simulink model "DatacenterUtilization"  (R2025b)
settings: Solver=daessc  StartTime=0.0  StopTime=7776000  FixedStep=3600  MaxStep=3600  RelTol=1e-3  AbsTol=1e-3
undefined symbols (not defined in the file or in its folder): Datacenter, MyDatacenterModelLib, Room
libraries: fl_lib x111, buildingEnergy_lib x13, datacenter_lib x12, nesl_utility x5
settings Model: Creator=vikrants  LastModifiedBy=skota
settings SolverCC: AutoScaleAbsTol=off  AlgebraicLoopSolver=TrustRegion  MaxZcPerStep=1.0
settings DataIOCC: SaveOutput=off  SignalLogging=off  DSMLogging=off  SaveTime=off  ReturnWorkspaceOutputs=off  TimeSaveName=tSim  SignalLoggingName=sglDatacenterUtilization  ReturnWorkspaceOutputsName=resDatacenterUtilization
settings DebuggingCC: UnconnectedInputMsg=warning  UnconnectedOutputMsg=warning  UnconnectedLineMsg=warning  SymbolicDimsDataTypeCodeGenerationDiagnostic=none
settings ModelReferenceCC: EnableRefExpFcnMdlSchedulingChecks=on
settings SFSimCC: CustomCodeUndefinedFunction=UseInterfaceOnly
settings RTWCC: GPUComputeCapability=3.5  DLArmComputeVersion=19.05
settings SimscapeCC: SimscapeLogType=all  SimscapeLogName=simlogDatacenterUtilization  SimscapeLogLimitData=off  SimscapeLogDataHistory=10000.0  SimscapeCompileComponentReuse=on

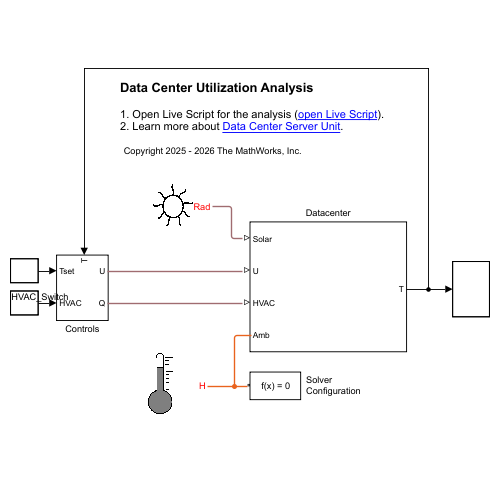
[thumbnail: Simulink's stored preview of the top-level diagram]
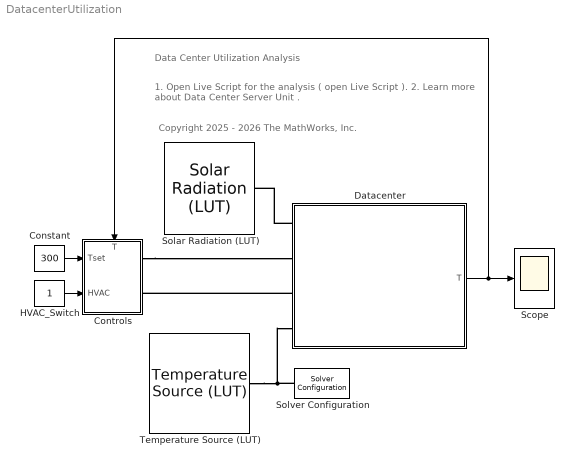
== system DatacenterUtilization ==
  note: Copyright 2025 - 2026 The MathWorks, Inc.
  note: Data Center Utilization Analysis
  note: 1. Open Live Script for the analysis ( open Live Script ).
      | 2. Learn more about Data Center Server Unit .
  Constant : Constant  Value=300
  Controls : Subsystem
      settings: PortSchema="{\"entries\":[{\"content\":{\"sides\":[{\"content\":{\"connectorIds\":[\"In1\",\"In2\"]},\"type\":\"ConnectorPlacement.EquallySpacedRectSide\",\"uuid\":\"920383aa-55f0-46ec-be25-1a0e41e599a9\"},{\"content\":{\"connectorIds\":[\"RConn1\",\"RConn2\"],\"side\":\"RIGHT\"},\"type\":\"ConnectorPlacement.EquallySpacedRectSide\",\"uuid\":\"2611bc07-e966-40b9-ba68-b41ec292afae\"},{\"content\":{\"connectorIds\":[\"In3\"],\"side\":\"TOP\"},\"type\":\"ConnectorPlacement.EquallySpacedRectSide\",\"uuid\":\"ac1e2822-ea25-44fd-bd61-5e24e36934cf\"}]},\"type\":\"ConnectorPlacement.EquallySpacedConnector\",\"uuid\":\"6950ab52-c187-4a89-be73-f973560319f4\"}],\"packageUris\":[\"http://schema.mathworks.com/mf0/Connector/R2020b\"],\"version\":\"1.0\"}"
  Datacenter : Subsystem
  HVAC_Switch : Constant
  Scope : Scope
      settings: ActiveDisplayYMinimum=298.50227589858127  ActiveDisplayYMaximum=313.47951691276859
  Solar Radiation (LUT) : buildingEnergy_lib/Solar Radiation (LUT)  latitude=12.971 % Parameterized on : 26-May-2026 12:20:46  longitude=77.594 % Parameterized on : 26-May-2026 12:20:46  localTime=82.5 % Parameterized on : 26-May-2026 12:20:46  dayLightS=0 % Parameterized on : 26-May-2026 12:20:46  startYear=2025 % Parameterized on : 26-May-2026 12:20:46  startMonth=1 % Parameterized on : 26-May-2026 12:20:46  startDay=1 % Parameterized on : 26-May-2026 12:20:46  startHr=1 % Parameterized on : 26-May-2026 12:20:46  numHrsData=2160 % Parameterized on : 26-May-2026 12:20:46  cloudData=cloudCoverLibOption.none  cloudCoverVal=zeros(1, 24)  interp_method=simscape.enum.interpolation.linear  extrap_method=simscape.enum.extrapolation.nearest
  Solver Configuration : nesl_utility/Solver Configuration  PhysicalDomain=network_engine_domain  SubClassName=solver  LeftPortType=input  RightPortType=generic  Tones=[]  Harmonics=[]  SimulateNoise=off  Profile=off  UseLocalSampling=off  EnableSwitchedLinearOptims=on  FrequencyDomain=off  UseCCode=off  RelTol=0.001  AbsTol=1e-06  MinStep=1e-09  ToWorkspace=off  RevertToSquareIcSolve=off  NumHomotopyIterations=100  PhasorMode=off  PhasorModeNumHarmonics=1  ConsistencySolver=NEWTON_XTOL_AFTER_FTOL  CanonicalOrdering=UNORDERED  OptimizeIntermediates=UNOPTIMIZED  IndexReductionMethod=DerivativeReplacement  DoDC=off  ResidualTolerance=1e-09  ConsistencyTolSource=GLOBAL  ConsistencyAbsTol=0.001  ConsistencyRelTol=0.001  ConsistencyTolFactor=0.001  UseLocalSolver=off  LocalSolverChoice=NE_BACKWARD_EULER_ADVANCER  ResolveIndetEquations=on  FunctionEvalNumThread=1  LocalSolverSampleTime=0.001  DoFixedCost=off  MaxNonlinIter=3  MaxModeIter=2  ComputeImpulses=off  ImpulseIterations=2  LinearAlgebra=auto  LinearAlgebraNumThread=0  EquationFormulation=NE_TIME_EF  DelaysMemoryBudget=1024  AutomaticFiltering=on  FilteringTimeConstant=0.001  PartitionStorageMethod=AS_NEEDED  PartitionMemoryBudget=1024  PartitionMethod=ROBUST  MultibodyUseLocalSolver=off  MultibodyLocalSolverChoice=ODE1  MultibodyLocalSolverSampleTime=0.001
  Temperature Source (LUT) : buildingEnergy_lib/Temperature Source (LUT)  latitude=12.971 % Parameterized on : 26-May-2026 12:20:45  longitude=77.594 % Parameterized on : 26-May-2026 12:20:45  localTime=82.5 % Parameterized on : 26-May-2026 12:20:45  dayLightS=0 % Parameterized on : 26-May-2026 12:20:46  startYear=2025 % Parameterized on : 26-May-2026 12:20:46  startMonth=1 % Parameterized on : 26-May-2026 12:20:46  startDay=1 % Parameterized on : 26-May-2026 12:20:46  startHr=1 % Parameterized on : 26-May-2026 12:20:46  numDaysData=91 % Parameterized on : 26-May-2026 12:20:46  interp_method=simscape.enum.interpolation.linear  extrap_method=simscape.enum.extrapolation.error  avgDayTvec=[309 309 309 309 309 309 309 309 309 309 309 309 309 309 309 309 309 309 309 309 309 309 309 309 309 309 309 309 309 309 309 309 309 309 309 309 309 309 309 309 309 309 309 309 309 309 309 309 309 309 309 309 309 309 309 309 309 309 309 309 309 309 309 309 309 309 309 309 309 309 309 309 309 309 309 309 309 309 309 309 309 309 309 309 309 309 309 309 309 309 309] K  pcDayTvar=5  avgNightTvec=[301 301 301 301 301 301 301 301 301 301 301 301 301 301 301 301 301 301 301 301 301 301 301 301 301 301 301 301 301 301 301 301 301 301 301 301 301 301 301 301 301 301 301 301 301 301 301 301 301 301 301 301 301 301 301 301 301 301 301 301 301 301 301 301 301 301 301 301 301 301 301 301 301 301 301 301 301 301 301 301 301 301 301 301 301 301 301 301 301 301 301] K  pcNightTvar=5
  wires:
  Constant/1 -> Controls/1(Tset)
  Datacenter/1(T) -> Scope/1, Controls/3(T)
  HVAC_Switch/1 -> Controls/2(HVAC)
  connections:
  Solver Configuration/RConn1 -- Temperature Source (LUT)/RConn1 -- Datacenter/LConn4
  Datacenter/LConn3 -- Controls/RConn2
  Datacenter/LConn1 -- Solar Radiation (LUT)/RConn1
  Controls/RConn1 -- Datacenter/LConn2

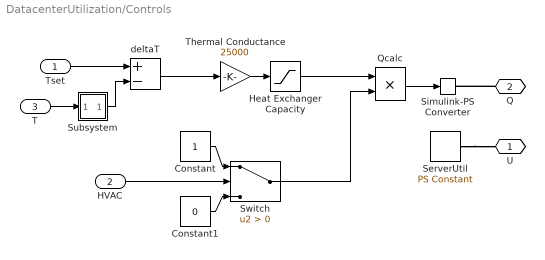
== system DatacenterUtilization/Controls ==
  Tset : Inport
  HVAC : Inport  Port=2
  T : Inport  Port=3
  Constant : Constant
  Constant1 : Constant  Value=0
  Heat Exchanger Capacity : Saturate  UpperLimit=100000  LowerLimit=-100000
  Qcalc : Product
  ServerUtil : fl_lib/Physical Signals/Sources/PS Constant  constant=[0.48 0.42 0.45 0.51 0.52 0.58 0.37 0.33 0.39 0.44 0.41 0.41]
  Simulink-PS Converter : nesl_utility/Simulink-PS Converter  PhysicalDomain=network_engine_domain  SubClassName=ps_input  LeftPortType=input  RightPortType=output  PseudoPeriodic=off  Frequencies=[]  NoiseDistribution=none  NoiseParameters=[]  Unit=W  AffineConversion=off  FilteringAndDerivatives=provide  SimscapeFilterOrder=1  InputFilterTimeConstant=0.001  UdotUserProvided=0
  Subsystem : Subsystem
  Switch : Switch  Criteria=u2 > Threshold  SaturateOnIntegerOverflow=off  InputSameDT=off
  Thermal Conductance : Gain  Gain=25000
  deltaT : Sum  Inputs=+-
  U : PMIOPort  Side=Right
  Q : PMIOPort  Port=2  Side=Right
  wires:
  Tset/1 -> deltaT/1
  HVAC/1 -> Switch/2
  Constant/1 -> Switch/1
  Constant1/1 -> Switch/3
  Switch/1 -> Qcalc/2
  Qcalc/1 -> Simulink-PS Converter/1
  deltaT/1 -> Thermal Conductance/1
  Thermal Conductance/1 -> Heat Exchanger Capacity/1
  Heat Exchanger Capacity/1 -> Qcalc/1
  T/1 -> Subsystem/1("  ")
  Subsystem/1(" ") -> deltaT/2
  connections:
  Q/RConn1 -- Simulink-PS Converter/RConn1
  ServerUtil/RConn1 -- U/RConn1

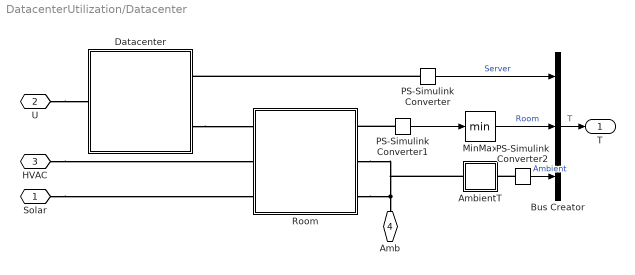
== system DatacenterUtilization/Datacenter ==
  AmbientT : Subsystem
  Bus Creator : BusCreator  Inputs=3
  Datacenter : Subsystem  AncestorBlock=MyDatacenterModelLib/Datacenter
  MinMax : MinMax
  PS-Simulink Converter : nesl_utility/PS-Simulink Converter  PhysicalDomain=network_engine_domain  SubClassName=ps_output  LeftPortType=input  RightPortType=output  PseudoPeriodic=off  Frequencies=[]  VectorFormat=inherit  Unit=inherit  AffineConversion=off
  PS-Simulink Converter1 : nesl_utility/PS-Simulink Converter  PhysicalDomain=network_engine_domain  SubClassName=ps_output  LeftPortType=input  RightPortType=output  PseudoPeriodic=off  Frequencies=[]  VectorFormat=inherit  Unit=inherit  AffineConversion=off
  PS-Simulink Converter2 : nesl_utility/PS-Simulink Converter  PhysicalDomain=network_engine_domain  SubClassName=ps_output  LeftPortType=input  RightPortType=output  PseudoPeriodic=off  Frequencies=[]  VectorFormat=inherit  Unit=inherit  AffineConversion=off
  Room : Subsystem  AncestorBlock=MyDatacenterModelLib/Room
  Solar : PMIOPort  Side=Left
  U : PMIOPort  Port=2  Side=Left
  HVAC : PMIOPort  Port=3  Side=Left
  Amb : PMIOPort  Port=4  Side=Left
  T : Outport
  wires:
  Bus Creator/1 -> T/1  "T"
  PS-Simulink Converter2/1 -> Bus Creator/3  "Ambient"
  PS-Simulink Converter1/1 -> MinMax/1
  PS-Simulink Converter/1 -> Bus Creator/1  "Server"
  MinMax/1 -> Bus Creator/2  "Room"
  connections:
  PS-Simulink Converter2/LConn1 -- AmbientT/RConn1
  Datacenter/RConn2 -- Room/LConn1
  U/RConn1 -- Datacenter/LConn1
  PS-Simulink Converter/LConn1 -- Datacenter/RConn1
  Room/RConn3 -- Room/RConn2 -- AmbientT/LConn1 -- Amb/RConn1
  PS-Simulink Converter1/LConn1 -- Room/RConn1
  HVAC/RConn1 -- Room/LConn2
  Solar/RConn1 -- Room/LConn3

== system DatacenterUtilization/Controls/Subsystem ==
  "  " : Inport
  Bus Selector1 : BusSelector  OutputSignals=Room
  Transfer Fcn : TransferFcn  Denominator=[1 1]
  " " : Outport
  wires:
  Bus Selector1/1 -> Transfer Fcn/1  "<Room>"
  "  "/1 -> Bus Selector1/1
  Transfer Fcn/1 -> " "/1

== system DatacenterUtilization/Datacenter/AmbientT ==
  Tref : fl_lib/Thermal/Thermal Elements/Thermal Reference
  Tsensor3 : fl_lib/Thermal/Thermal Sensors/Temperature Sensor  temperature_measure=foundation.enum.MeasurementReference.difference
  "   " : PMIOPort  Side=Left
  T : PMIOPort  Port=2  Side=Right
  connections:
  Tsensor3/RConn1 -- Tref/LConn1
  Tsensor3/RConn2 -- T/RConn1
  Tsensor3/LConn1 -- "   "/RConn1

== system DatacenterUtilization/Datacenter/Datacenter ==
  ServerUnits : Subsystem
  Util : PMIOPort  Side=Left
  T : PMIOPort  Port=2  Side=Right
  H : PMIOPort  Port=3  Side=Right
  connections:
  ServerUnits/RConn1 -- H/RConn1
  ServerUnits/RConn2 -- T/RConn1
  ServerUnits/LConn1 -- Util/RConn1

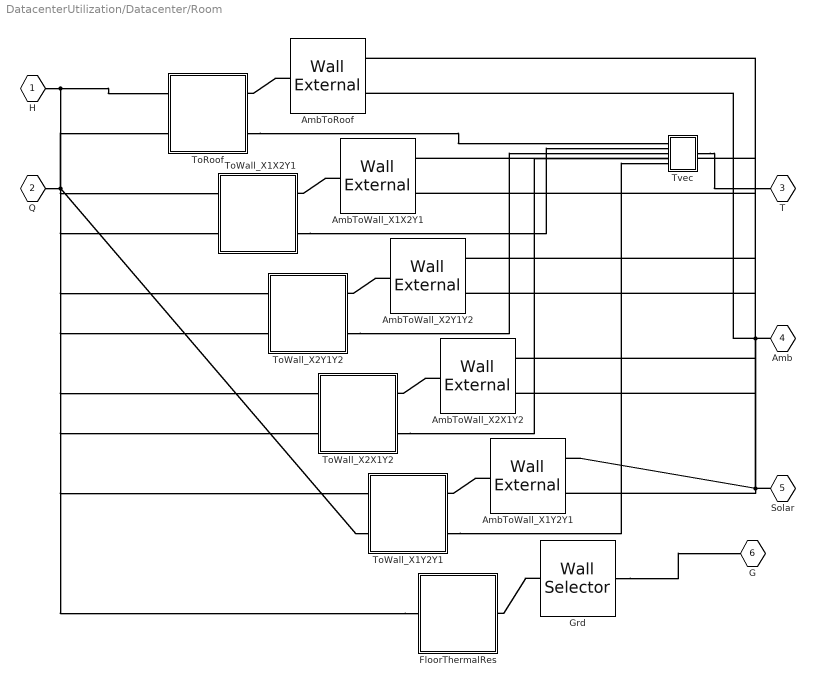
== system DatacenterUtilization/Datacenter/Room ==
  AmbToRoof : buildingEnergy_lib/Wall External  extWallModel=wallExternalModelOption.wallSolarWinVent  wallLength=12 m  wallHeight=8 m  wallThickness=0.05 m  wallMaterialDen=4000 kg/m^3  wallMaterialCp=1870 J/(K*kg)  wallAbsorptivity=0.5  wallThermalK=2 W/(K*m)  winLength=1 m  winHeight=0.5 m  winThickness=0.007 m  winMaterialDen=2500 kg/m^3  winMaterialCp=787 J/(K*kg)  winAbsorptivity=0.35  winThermalK=1 W/(K*m)  winTransmissivity=0.45  ventLength=0.1 m  ventHeight=0.1 m  extToWallHTC=5 W/(K*m^2)  intToRoomHTC=5 W/(K*m^2)  iniT=300 K  latitude=12.971 % Parameterized on : 26-May-2026 12:20:46  longitude=77.594 % Parameterized on : 26-May-2026 12:20:46  localTime=82.5 % Parameterized on : 26-May-2026 12:20:46  dayLightS=0 % Parameterized on : 26-May-2026 12:20:46  surfAngle=0 deg  surfUnitV="[0.42262    -0.90631]"  startYear=2025 % Parameterized on : 26-May-2026 12:20:46  startMonth=1 % Parameterized on : 26-May-2026 12:20:46  startDay=1 % Parameterized on : 26-May-2026 12:20:46  startHr=1 % Parameterized on : 26-May-2026 12:20:46  numHrsData=2160 % Parameterized on : 26-May-2026 12:20:46  interp_method=simscape.enum.interpolation.linear  extrap_method=simscape.enum.extrapolation.nearest
  AmbToWall_X1X2Y1 : buildingEnergy_lib/Wall External  extWallModel=wallExternalModelOption.wallSolarWinVent  wallLength=12 m  wallHeight=3 m  wallThickness=0.05 m  wallMaterialDen=4000 kg/m^3  wallMaterialCp=1870 J/(K*kg)  wallAbsorptivity=0.5  wallThermalK=2 W/(K*m)  winLength=1 m  winHeight=0.5 m  winThickness=0.007 m  winMaterialDen=2500 kg/m^3  winMaterialCp=787 J/(K*kg)  winAbsorptivity=0.35  winThermalK=1 W/(K*m)  winTransmissivity=0.45  ventLength=0.1 m  ventHeight=0.1 m  extToWallHTC=5 W/(K*m^2)  intToRoomHTC=5 W/(K*m^2)  iniT=300 K  latitude=12.971 % Parameterized on : 26-May-2026 12:20:46  longitude=77.594 % Parameterized on : 26-May-2026 12:20:46  localTime=82.5 % Parameterized on : 26-May-2026 12:20:46  dayLightS=0 % Parameterized on : 26-May-2026 12:20:46  surfAngle=90 deg  surfUnitV="[0.42262    -0.90631]"  startYear=2025 % Parameterized on : 26-May-2026 12:20:46  startMonth=1 % Parameterized on : 26-May-2026 12:20:46  startDay=1 % Parameterized on : 26-May-2026 12:20:46  startHr=1 % Parameterized on : 26-May-2026 12:20:46  numHrsData=2160 % Parameterized on : 26-May-2026 12:20:46  interp_method=simscape.enum.interpolation.linear  extrap_method=simscape.enum.extrapolation.nearest
  AmbToWall_X1Y2Y1 : buildingEnergy_lib/Wall External  extWallModel=wallExternalModelOption.wallSolarWinVent  wallLength=8 m  wallHeight=3 m  wallThickness=0.05 m  wallMaterialDen=4000 kg/m^3  wallMaterialCp=1870 J/(K*kg)  wallAbsorptivity=0.5  wallThermalK=2 W/(K*m)  winLength=1 m  winHeight=0.5 m  winThickness=0.007 m  winMaterialDen=2500 kg/m^3  winMaterialCp=787 J/(K*kg)  winAbsorptivity=0.35  winThermalK=1 W/(K*m)  winTransmissivity=0.45  ventLength=0.1 m  ventHeight=0.1 m  extToWallHTC=5 W/(K*m^2)  intToRoomHTC=5 W/(K*m^2)  iniT=300 K  latitude=12.971 % Parameterized on : 26-May-2026 12:20:46  longitude=77.594 % Parameterized on : 26-May-2026 12:20:46  localTime=82.5 % Parameterized on : 26-May-2026 12:20:46  dayLightS=0 % Parameterized on : 26-May-2026 12:20:46  surfAngle=90 deg  surfUnitV="[-0.90631    -0.42262]"  startYear=2025 % Parameterized on : 26-May-2026 12:20:46  startMonth=1 % Parameterized on : 26-May-2026 12:20:46  startDay=1 % Parameterized on : 26-May-2026 12:20:46  startHr=1 % Parameterized on : 26-May-2026 12:20:46  numHrsData=2160 % Parameterized on : 26-May-2026 12:20:46  interp_method=simscape.enum.interpolation.linear  extrap_method=simscape.enum.extrapolation.nearest
  AmbToWall_X2X1Y2 : buildingEnergy_lib/Wall External  extWallModel=wallExternalModelOption.wallSolarWinVent  wallLength=12 m  wallHeight=3 m  wallThickness=0.05 m  wallMaterialDen=4000 kg/m^3  wallMaterialCp=1870 J/(K*kg)  wallAbsorptivity=0.5  wallThermalK=2 W/(K*m)  winLength=1 m  winHeight=0.5 m  winThickness=0.007 m  winMaterialDen=2500 kg/m^3  winMaterialCp=787 J/(K*kg)  winAbsorptivity=0.35  winThermalK=1 W/(K*m)  winTransmissivity=0.45  ventLength=0.1 m  ventHeight=0.1 m  extToWallHTC=5 W/(K*m^2)  intToRoomHTC=5 W/(K*m^2)  iniT=300 K  latitude=12.971 % Parameterized on : 26-May-2026 12:20:46  longitude=77.594 % Parameterized on : 26-May-2026 12:20:46  localTime=82.5 % Parameterized on : 26-May-2026 12:20:46  dayLightS=0 % Parameterized on : 26-May-2026 12:20:46  surfAngle=90 deg  surfUnitV="[-0.42262     0.90631]"  startYear=2025 % Parameterized on : 26-May-2026 12:20:46  startMonth=1 % Parameterized on : 26-May-2026 12:20:46  startDay=1 % Parameterized on : 26-May-2026 12:20:46  startHr=1 % Parameterized on : 26-May-2026 12:20:46  numHrsData=2160 % Parameterized on : 26-May-2026 12:20:46  interp_method=simscape.enum.interpolation.linear  extrap_method=simscape.enum.extrapolation.nearest
  AmbToWall_X2Y1Y2 : buildingEnergy_lib/Wall External  extWallModel=wallExternalModelOption.wallSolarWinVent  wallLength=8 m  wallHeight=3 m  wallThickness=0.05 m  wallMaterialDen=4000 kg/m^3  wallMaterialCp=1870 J/(K*kg)  wallAbsorptivity=0.5  wallThermalK=2 W/(K*m)  winLength=1 m  winHeight=0.5 m  winThickness=0.007 m  winMaterialDen=2500 kg/m^3  winMaterialCp=787 J/(K*kg)  winAbsorptivity=0.35  winThermalK=1 W/(K*m)  winTransmissivity=0.45  ventLength=0.1 m  ventHeight=0.1 m  extToWallHTC=5 W/(K*m^2)  intToRoomHTC=5 W/(K*m^2)  iniT=300 K  latitude=12.971 % Parameterized on : 26-May-2026 12:20:46  longitude=77.594 % Parameterized on : 26-May-2026 12:20:46  localTime=82.5 % Parameterized on : 26-May-2026 12:20:46  dayLightS=0 % Parameterized on : 26-May-2026 12:20:46  surfAngle=90 deg  surfUnitV="[0.90631     0.42262]"  startYear=2025 % Parameterized on : 26-May-2026 12:20:46  startMonth=1 % Parameterized on : 26-May-2026 12:20:46  startDay=1 % Parameterized on : 26-May-2026 12:20:46  startHr=1 % Parameterized on : 26-May-2026 12:20:46  numHrsData=2160 % Parameterized on : 26-May-2026 12:20:46  interp_method=simscape.enum.interpolation.linear  extrap_method=simscape.enum.extrapolation.nearest
  FloorThermalRes : Subsystem
  Grd : buildingEnergy_lib/Wall Selector  optWall=1  wallLength=12 m  wallHeight=8 m  wallThickness=0.05 m  wallMaterialDen=4000 kg/m^3  wallMaterialCp=1870 J/(K*kg)  wallAbsorptivity=0.5  wallThermalK=2 W/(K*m)  winLength=1 m  winHeight=0.5 m  winThickness=0.007 m  winMaterialDen=2500 kg/m^3  winMaterialCp=787 J/(K*kg)  winAbsorptivity=0.35  winThermalK=1 W/(K*m)  winTransmissivity=0.45  ventLength=0.1 m  ventHeight=0.1 m  extToWallHTC=5 W/(K*m^2)  intToRoomHTC=5 W/(K*m^2)  iniT=300 K
  ToRoof : Subsystem
  ToWall_X1X2Y1 : Subsystem
  ToWall_X1Y2Y1 : Subsystem
  ToWall_X2X1Y2 : Subsystem
  ToWall_X2Y1Y2 : Subsystem
  Tvec : Subsystem
  H : PMIOPort  Side=Left
  Q : PMIOPort  Port=2  Side=Left
  T : PMIOPort  Port=3  Side=Right
  Amb : PMIOPort  Port=4  Side=Right
  Solar : PMIOPort  Port=5  Side=Left
  G : PMIOPort  Port=6  Side=Right
  connections:
  Grd/RConn1 -- FloorThermalRes/RConn1
  Grd/LConn1 -- G/RConn1
  Tvec/RConn1 -- T/RConn1
  ToWall_X1Y2Y1/RConn2 -- Tvec/LConn5
  AmbToWall_X1Y2Y1/RConn1 -- ToWall_X1Y2Y1/RConn1
  ToWall_X2X1Y2/RConn2 -- Tvec/LConn4
  AmbToWall_X2X1Y2/RConn1 -- ToWall_X2X1Y2/RConn1
  ToWall_X2Y1Y2/RConn2 -- Tvec/LConn3
  AmbToWall_X2Y1Y2/RConn1 -- ToWall_X2Y1Y2/RConn1
  ToWall_X1X2Y1/RConn2 -- Tvec/LConn2
  AmbToWall_X1X2Y1/RConn1 -- ToWall_X1X2Y1/RConn1
  ToRoof/RConn2 -- Tvec/LConn1
  AmbToWall_X1Y2Y1/LConn1 -- AmbToWall_X2X1Y2/LConn1 -- AmbToWall_X2Y1Y2/LConn1 -- AmbToWall_X1X2Y1/LConn1 -- Solar/RConn1 -- AmbToRoof/LConn1
  AmbToWall_X1Y2Y1/LConn2 -- AmbToWall_X2X1Y2/LConn2 -- AmbToWall_X2Y1Y2/LConn2 -- AmbToWall_X1X2Y1/LConn2 -- Amb/RConn1 -- AmbToRoof/LConn2
  AmbToRoof/RConn1 -- ToRoof/RConn1
  ToWall_X1Y2Y1/LConn2 -- ToWall_X2X1Y2/LConn2 -- ToWall_X2Y1Y2/LConn2 -- ToWall_X1X2Y1/LConn2 -- Q/RConn1 -- ToRoof/LConn2
  FloorThermalRes/LConn1 -- ToWall_X1Y2Y1/LConn1 -- ToWall_X2X1Y2/LConn1 -- ToWall_X2Y1Y2/LConn1 -- ToWall_X1X2Y1/LConn1 -- H/RConn1 -- ToRoof/LConn1

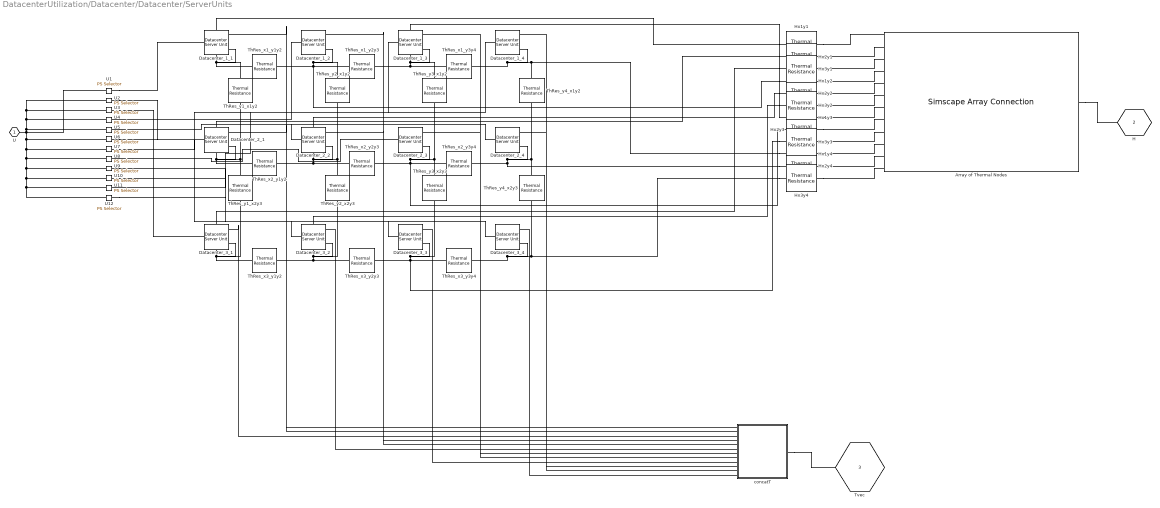
== system DatacenterUtilization/Datacenter/Datacenter/ServerUnits ==
  Array of Thermal Nodes : SimscapeArrayConnection  Domain=foundation.thermal.thermal  ConcatenateDimension=1  NumScalarElements=12
  Datacenter_1_{1..4} (4 alike) : datacenter_lib/Datacenter Server Unit  peakPowCPU=40 W  numOfCPU=2  peakPowMemory=9 W  numOfMemory=4  peakPowDisk=12 W  numOfDisk=1  peakPowPCIslot=25 W  numOfPCIslot=2  peakPowMotherboard=25 W  numOfMotherboard=1  peakPowFan=10 W  numOfFan=1  powerSupplyEff=85  numCPUperServer=11  ratioActualToNameplate=0.6  serverMass=50 kg  serverSpHeat=2500 J/(K*kg)  idlePower=25 W  physQ=datacenterPhysics.linear  calibParam=1  T_specify=off  T_priority=High  T=300 K  T_nominal_specify=off  T_nominal_value=1  T_nominal_unit=K  Q_specify=off  Q_priority=None  Q=0 W  Q_nominal_specify=off  Q_nominal_value=1  Q_nominal_unit=W
  Datacenter_2_{1..4} (4 alike) : datacenter_lib/Datacenter Server Unit  peakPowCPU=40 W  numOfCPU=2  peakPowMemory=9 W  numOfMemory=4  peakPowDisk=12 W  numOfDisk=1  peakPowPCIslot=25 W  numOfPCIslot=2  peakPowMotherboard=25 W  numOfMotherboard=1  peakPowFan=10 W  numOfFan=1  powerSupplyEff=85  numCPUperServer=11  ratioActualToNameplate=0.6  serverMass=50 kg  serverSpHeat=2500 J/(K*kg)  idlePower=25 W  physQ=datacenterPhysics.linear  calibParam=1  T_specify=off  T_priority=High  T=300 K  T_nominal_specify=off  T_nominal_value=1  T_nominal_unit=K  Q_specify=off  Q_priority=None  Q=0 W  Q_nominal_specify=off  Q_nominal_value=1  Q_nominal_unit=W
  Datacenter_3_{1..4} (4 alike) : datacenter_lib/Datacenter Server Unit  peakPowCPU=40 W  numOfCPU=2  peakPowMemory=9 W  numOfMemory=4  peakPowDisk=12 W  numOfDisk=1  peakPowPCIslot=25 W  numOfPCIslot=2  peakPowMotherboard=25 W  numOfMotherboard=1  peakPowFan=10 W  numOfFan=1  powerSupplyEff=85  numCPUperServer=11  ratioActualToNameplate=0.6  serverMass=50 kg  serverSpHeat=2500 J/(K*kg)  idlePower=25 W  physQ=datacenterPhysics.linear  calibParam=1  T_specify=off  T_priority=High  T=300 K  T_nominal_specify=off  T_nominal_value=1  T_nominal_unit=K  Q_specify=off  Q_priority=None  Q=0 W  Q_nominal_specify=off  Q_nominal_value=1  Q_nominal_unit=W
  Hx1y{1..4} (4 alike) : fl_lib/Thermal/Thermal Elements/Thermal Resistance  resistance=0.01 K/W  T_specify=off  T_priority=None  T=0 K  T_nominal_specify=off  T_nominal_value=1  T_nominal_unit=K  Q_specify=off  Q_priority=None  Q=0 W  Q_nominal_specify=off  Q_nominal_value=1  Q_nominal_unit=W
  Hx2y{1..4} (4 alike) : fl_lib/Thermal/Thermal Elements/Thermal Resistance  resistance=0.01 K/W  T_specify=off  T_priority=None  T=0 K  T_nominal_specify=off  T_nominal_value=1  T_nominal_unit=K  Q_specify=off  Q_priority=None  Q=0 W  Q_nominal_specify=off  Q_nominal_value=1  Q_nominal_unit=W
  Hx3y{1..4} (4 alike) : fl_lib/Thermal/Thermal Elements/Thermal Resistance  resistance=0.01 K/W  T_specify=off  T_priority=None  T=0 K  T_nominal_specify=off  T_nominal_value=1  T_nominal_unit=K  Q_specify=off  Q_priority=None  Q=0 W  Q_nominal_specify=off  Q_nominal_value=1  Q_nominal_unit=W
  ThRes_x1_y1y2 : fl_lib/Thermal/Thermal Elements/Thermal Resistance  resistance=0.01 K/W  T_specify=off  T_priority=None  T=0 K  T_nominal_specify=off  T_nominal_value=1  T_nominal_unit=K  Q_specify=off  Q_priority=None  Q=0 W  Q_nominal_specify=off  Q_nominal_value=1  Q_nominal_unit=W
  ThRes_x1_y2y3 : fl_lib/Thermal/Thermal Elements/Thermal Resistance  resistance=0.01 K/W  T_specify=off  T_priority=None  T=0 K  T_nominal_specify=off  T_nominal_value=1  T_nominal_unit=K  Q_specify=off  Q_priority=None  Q=0 W  Q_nominal_specify=off  Q_nominal_value=1  Q_nominal_unit=W
  ThRes_x1_y3y4 : fl_lib/Thermal/Thermal Elements/Thermal Resistance  resistance=0.01 K/W  T_specify=off  T_priority=None  T=0 K  T_nominal_specify=off  T_nominal_value=1  T_nominal_unit=K  Q_specify=off  Q_priority=None  Q=0 W  Q_nominal_specify=off  Q_nominal_value=1  Q_nominal_unit=W
  ThRes_x2_y1y2 : fl_lib/Thermal/Thermal Elements/Thermal Resistance  resistance=0.01 K/W  T_specify=off  T_priority=None  T=0 K  T_nominal_specify=off  T_nominal_value=1  T_nominal_unit=K  Q_specify=off  Q_priority=None  Q=0 W  Q_nominal_specify=off  Q_nominal_value=1  Q_nominal_unit=W
  ThRes_x2_y2y3 : fl_lib/Thermal/Thermal Elements/Thermal Resistance  resistance=0.01 K/W  T_specify=off  T_priority=None  T=0 K  T_nominal_specify=off  T_nominal_value=1  T_nominal_unit=K  Q_specify=off  Q_priority=None  Q=0 W  Q_nominal_specify=off  Q_nominal_value=1  Q_nominal_unit=W
  ThRes_x2_y3y4 : fl_lib/Thermal/Thermal Elements/Thermal Resistance  resistance=0.01 K/W  T_specify=off  T_priority=None  T=0 K  T_nominal_specify=off  T_nominal_value=1  T_nominal_unit=K  Q_specify=off  Q_priority=None  Q=0 W  Q_nominal_specify=off  Q_nominal_value=1  Q_nominal_unit=W
  ThRes_x3_y1y2 : fl_lib/Thermal/Thermal Elements/Thermal Resistance  resistance=0.01 K/W  T_specify=off  T_priority=None  T=0 K  T_nominal_specify=off  T_nominal_value=1  T_nominal_unit=K  Q_specify=off  Q_priority=None  Q=0 W  Q_nominal_specify=off  Q_nominal_value=1  Q_nominal_unit=W
  ThRes_x3_y2y3 : fl_lib/Thermal/Thermal Elements/Thermal Resistance  resistance=0.01 K/W  T_specify=off  T_priority=None  T=0 K  T_nominal_specify=off  T_nominal_value=1  T_nominal_unit=K  Q_specify=off  Q_priority=None  Q=0 W  Q_nominal_specify=off  Q_nominal_value=1  Q_nominal_unit=W
  ThRes_x3_y3y4 : fl_lib/Thermal/Thermal Elements/Thermal Resistance  resistance=0.01 K/W  T_specify=off  T_priority=None  T=0 K  T_nominal_specify=off  T_nominal_value=1  T_nominal_unit=K  Q_specify=off  Q_priority=None  Q=0 W  Q_nominal_specify=off  Q_nominal_value=1  Q_nominal_unit=W
  ThRes_y1_x1y2 : fl_lib/Thermal/Thermal Elements/Thermal Resistance  resistance=0.01 K/W  T_specify=off  T_priority=None  T=0 K  T_nominal_specify=off  T_nominal_value=1  T_nominal_unit=K  Q_specify=off  Q_priority=None  Q=0 W  Q_nominal_specify=off  Q_nominal_value=1  Q_nominal_unit=W
  ThRes_y1_x2y3 : fl_lib/Thermal/Thermal Elements/Thermal Resistance  resistance=0.01 K/W  T_specify=off  T_priority=None  T=0 K  T_nominal_specify=off  T_nominal_value=1  T_nominal_unit=K  Q_specify=off  Q_priority=None  Q=0 W  Q_nominal_specify=off  Q_nominal_value=1  Q_nominal_unit=W
  ThRes_y2_x1y2 : fl_lib/Thermal/Thermal Elements/Thermal Resistance  resistance=0.01 K/W  T_specify=off  T_priority=None  T=0 K  T_nominal_specify=off  T_nominal_value=1  T_nominal_unit=K  Q_specify=off  Q_priority=None  Q=0 W  Q_nominal_specify=off  Q_nominal_value=1  Q_nominal_unit=W
  ThRes_y2_x2y3 : fl_lib/Thermal/Thermal Elements/Thermal Resistance  resistance=0.01 K/W  T_specify=off  T_priority=None  T=0 K  T_nominal_specify=off  T_nominal_value=1  T_nominal_unit=K  Q_specify=off  Q_priority=None  Q=0 W  Q_nominal_specify=off  Q_nominal_value=1  Q_nominal_unit=W
  ThRes_y3_x1y2 : fl_lib/Thermal/Thermal Elements/Thermal Resistance  resistance=0.01 K/W  T_specify=off  T_priority=None  T=0 K  T_nominal_specify=off  T_nominal_value=1  T_nominal_unit=K  Q_specify=off  Q_priority=None  Q=0 W  Q_nominal_specify=off  Q_nominal_value=1  Q_nominal_unit=W
  ThRes_y3_x2y3 : fl_lib/Thermal/Thermal Elements/Thermal Resistance  resistance=0.01 K/W  T_specify=off  T_priority=None  T=0 K  T_nominal_specify=off  T_nominal_value=1  T_nominal_unit=K  Q_specify=off  Q_priority=None  Q=0 W  Q_nominal_specify=off  Q_nominal_value=1  Q_nominal_unit=W
  ThRes_y4_x1y2 : fl_lib/Thermal/Thermal Elements/Thermal Resistance  resistance=0.01 K/W  T_specify=off  T_priority=None  T=0 K  T_nominal_specify=off  T_nominal_value=1  T_nominal_unit=K  Q_specify=off  Q_priority=None  Q=0 W  Q_nominal_specify=off  Q_nominal_value=1  Q_nominal_unit=W
  ThRes_y4_x2y3 : fl_lib/Thermal/Thermal Elements/Thermal Resistance  resistance=0.01 K/W  T_specify=off  T_priority=None  T=0 K  T_nominal_specify=off  T_nominal_value=1  T_nominal_unit=K  Q_specify=off  Q_priority=None  Q=0 W  Q_nominal_specify=off  Q_nominal_value=1  Q_nominal_unit=W
  U1 : fl_lib/Physical Signals/Nonlinear Operators/PS Selector  ix=1
  U10 : fl_lib/Physical Signals/Nonlinear Operators/PS Selector  ix=10
  U11 : fl_lib/Physical Signals/Nonlinear Operators/PS Selector  ix=11
  U12 : fl_lib/Physical Signals/Nonlinear Operators/PS Selector  ix=12
  U2 : fl_lib/Physical Signals/Nonlinear Operators/PS Selector  ix=2
  U3 : fl_lib/Physical Signals/Nonlinear Operators/PS Selector  ix=3
  U4 : fl_lib/Physical Signals/Nonlinear Operators/PS Selector  ix=4
  U5 : fl_lib/Physical Signals/Nonlinear Operators/PS Selector  ix=5
  U6 : fl_lib/Physical Signals/Nonlinear Operators/PS Selector  ix=6
  U7 : fl_lib/Physical Signals/Nonlinear Operators/PS Selector  ix=7
  U8 : fl_lib/Physical Signals/Nonlinear Operators/PS Selector  ix=8
  U9 : fl_lib/Physical Signals/Nonlinear Operators/PS Selector  ix=9
  concatT : Subsystem
  U : PMIOPort  Side=Left
  H : PMIOPort  Port=2  Side=Right
  Tvec : PMIOPort  Port=3  Side=Right
  connections:
  concatT/LConn12 -- Datacenter_3_4/RConn1
  concatT/LConn11 -- Datacenter_2_4/RConn1
  concatT/LConn10 -- Datacenter_1_4/RConn1
  concatT/LConn9 -- Datacenter_3_3/RConn1
  concatT/LConn8 -- Datacenter_2_3/RConn1
  concatT/LConn7 -- Datacenter_1_3/RConn1
  concatT/LConn6 -- Datacenter_3_2/RConn1
  concatT/LConn5 -- Datacenter_2_2/RConn1
  concatT/LConn4 -- Datacenter_1_2/RConn1
  concatT/LConn3 -- Datacenter_3_1/RConn1
  concatT/LConn2 -- Datacenter_2_1/RConn1
  concatT/LConn1 -- Datacenter_1_1/RConn1
  concatT/RConn1 -- Tvec/RConn1
  Hx3y4/RConn1 -- Array of Thermal Nodes/LConn12
  Hx2y4/RConn1 -- Array of Thermal Nodes/LConn11
  Hx1y4/RConn1 -- Array of Thermal Nodes/LConn10
  Hx3y3/RConn1 -- Array of Thermal Nodes/LConn9
  Hx2y3/RConn1 -- Array of Thermal Nodes/LConn8
  Hx1y3/RConn1 -- Array of Thermal Nodes/LConn7
  Hx3y2/RConn1 -- Array of Thermal Nodes/LConn6
  Hx2y2/RConn1 -- Array of Thermal Nodes/LConn5
  Hx1y2/RConn1 -- Array of Thermal Nodes/LConn4
  Hx3y1/RConn1 -- Array of Thermal Nodes/LConn3
  Hx2y1/RConn1 -- Array of Thermal Nodes/LConn2
  Hx1y1/RConn1 -- Array of Thermal Nodes/LConn1
  Array of Thermal Nodes/RConn1 -- H/RConn1
  U12/RConn1 -- Datacenter_3_4/LConn1
  U11/RConn1 -- Datacenter_2_4/LConn1
  U10/RConn1 -- Datacenter_1_4/LConn1
  U9/RConn1 -- Datacenter_3_3/LConn1
  U8/RConn1 -- Datacenter_2_3/LConn1
  U7/RConn1 -- Datacenter_1_3/LConn1
  U6/RConn1 -- Datacenter_3_2/LConn1
  U5/RConn1 -- Datacenter_2_2/LConn1
  U4/RConn1 -- Datacenter_1_2/LConn1
  U3/RConn1 -- Datacenter_3_1/LConn1
  U2/RConn1 -- Datacenter_2_1/LConn1
  U1/RConn1 -- Datacenter_1_1/LConn1
  U12/LConn1 -- U3/LConn1 -- U2/LConn1 -- U4/LConn1 -- U5/LConn1 -- U/RConn1 -- U1/LConn1 -- U6/LConn1 -- U7/LConn1 -- U8/LConn1 -- U9/LConn1 -- U10/LConn1 -- U11/LConn1
  Hx3y4/LConn1 -- Datacenter_3_4/RConn3 -- ThRes_x3_y3y4/RConn1 -- ThRes_y4_x2y3/RConn1
  Hx3y3/LConn1 -- ThRes_y3_x2y3/RConn1 -- Datacenter_3_3/RConn3 -- ThRes_x3_y3y4/LConn1 -- ThRes_x3_y2y3/RConn1
  Hx3y2/LConn1 -- ThRes_x3_y2y3/LConn1 -- ThRes_x3_y1y2/RConn1 -- ThRes_y2_x2y3/RConn1 -- Datacenter_3_2/RConn3
  Hx3y1/LConn1 -- ThRes_y1_x2y3/RConn1 -- Datacenter_3_1/RConn3 -- ThRes_x3_y1y2/LConn1
  Hx2y4/LConn1 -- ThRes_y4_x2y3/LConn1 -- ThRes_y4_x1y2/RConn1 -- Datacenter_2_4/RConn3 -- ThRes_x2_y3y4/RConn1
  Hx2y3/LConn1 -- ThRes_y3_x2y3/LConn1 -- ThRes_y3_x1y2/RConn1 -- Datacenter_2_3/RConn3 -- ThRes_x2_y3y4/LConn1 -- ThRes_x2_y2y3/RConn1
  Hx2y2/LConn1 -- ThRes_x2_y2y3/LConn1 -- ThRes_x2_y1y2/RConn1 -- ThRes_y2_x2y3/LConn1 -- ThRes_y2_x1y2/RConn1 -- Datacenter_2_2/RConn3
  Hx2y1/LConn1 -- ThRes_y1_x2y3/LConn1 -- ThRes_y1_x1y2/RConn1 -- Datacenter_2_1/RConn3 -- ThRes_x2_y1y2/LConn1
  Hx1y4/LConn1 -- Datacenter_1_4/RConn3 -- ThRes_x1_y3y4/RConn1 -- ThRes_y4_x1y2/LConn1
  Hx1y3/LConn1 -- ThRes_x1_y3y4/LConn1 -- ThRes_x1_y2y3/RConn1 -- ThRes_y3_x1y2/LConn1 -- Datacenter_1_3/RConn3
  Hx1y2/LConn1 -- ThRes_y2_x1y2/LConn1 -- Datacenter_1_2/RConn3 -- ThRes_x1_y2y3/LConn1 -- ThRes_x1_y1y2/RConn1
  Hx1y1/LConn1 -- ThRes_y1_x1y2/LConn1 -- Datacenter_1_1/RConn3 -- ThRes_x1_y1y2/LConn1

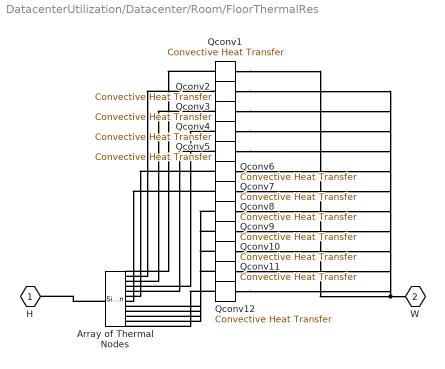
== system DatacenterUtilization/Datacenter/Room/FloorThermalRes ==
  Array of Thermal Nodes : SimscapeArrayConnection  Domain=foundation.thermal.thermal  ConcatenateDimension=1  NumScalarElements=12
  Qconv{1..12} (12 alike) : fl_lib/Thermal/Thermal Elements/Convective Heat Transfer  thermal_type=foundation.enum.constant_variable.constant  area=8 m^2  heat_tr_coeff=20 W/(K*m^2)  min_heat_tr_coeff=1e-3 W/(K*m^2)  T_specify=off  T_priority=None  T=0 K  T_nominal_specify=off  T_nominal_value=1  T_nominal_unit=K  Q_specify=off  Q_priority=None  Q=0 W  Q_nominal_specify=off  Q_nominal_value=1  Q_nominal_unit=W
  H : PMIOPort  Side=Left
  W : PMIOPort  Port=2  Side=Right
  connections:
  Qconv12/LConn1 -- Array of Thermal Nodes/LConn12
  Qconv11/LConn1 -- Array of Thermal Nodes/LConn11
  Qconv10/LConn1 -- Array of Thermal Nodes/LConn10
  Qconv9/LConn1 -- Array of Thermal Nodes/LConn9
  Qconv8/LConn1 -- Array of Thermal Nodes/LConn8
  Qconv7/LConn1 -- Array of Thermal Nodes/LConn7
  Qconv6/LConn1 -- Array of Thermal Nodes/LConn6
  Qconv5/LConn1 -- Array of Thermal Nodes/LConn5
  Qconv4/LConn1 -- Array of Thermal Nodes/LConn4
  Qconv3/LConn1 -- Array of Thermal Nodes/LConn3
  Qconv2/LConn1 -- Array of Thermal Nodes/LConn2
  Qconv12/RConn1 -- W/RConn1 -- Qconv11/RConn1 -- Qconv10/RConn1 -- Qconv9/RConn1 -- Qconv8/RConn1 -- Qconv7/RConn1 -- Qconv6/RConn1 -- Qconv5/RConn1 -- Qconv4/RConn1 -- Qconv3/RConn1 -- Qconv2/RConn1 -- Qconv1/RConn1
  Qconv1/LConn1 -- Array of Thermal Nodes/LConn1
  Array of Thermal Nodes/RConn1 -- H/RConn1

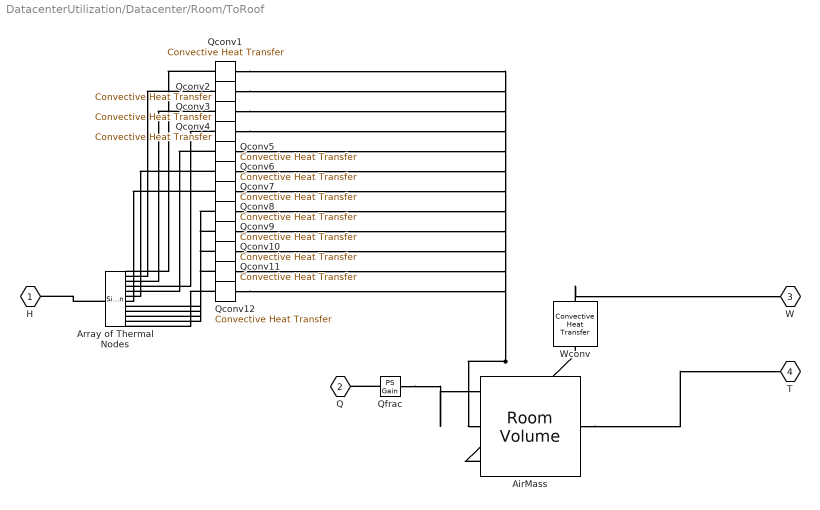
== system DatacenterUtilization/Datacenter/Room/ToRoof ==
  AirMass : buildingEnergy_lib/Room Volume  N1=1  N2=1  iniT=300 K  length=12 m  width=8 m  height=0.10667 m
  Array of Thermal Nodes : SimscapeArrayConnection  Domain=foundation.thermal.thermal  ConcatenateDimension=1  NumScalarElements=12
  Qconv{1..12} (12 alike) : fl_lib/Thermal/Thermal Elements/Convective Heat Transfer  thermal_type=foundation.enum.constant_variable.constant  area=8 m^2  heat_tr_coeff=20 W/(K*m^2)  min_heat_tr_coeff=1e-3 W/(K*m^2)  T_specify=off  T_priority=None  T=0 K  T_nominal_specify=off  T_nominal_value=1  T_nominal_unit=K  Q_specify=off  Q_priority=None  Q=0 W  Q_nominal_specify=off  Q_nominal_value=1  Q_nominal_unit=W
  Qfrac : fl_lib/Physical Signals/Functions/PS Gain  gain=0.44444
  Wconv : fl_lib/Thermal/Thermal Elements/Convective Heat Transfer  thermal_type=foundation.enum.constant_variable.constant  area=96 m^2  heat_tr_coeff=20 W/(K*m^2)  min_heat_tr_coeff=1e-3 W/(K*m^2)  T_specify=off  T_priority=None  T=0 K  T_nominal_specify=off  T_nominal_value=1  T_nominal_unit=K  Q_specify=off  Q_priority=None  Q=0 W  Q_nominal_specify=off  Q_nominal_value=1  Q_nominal_unit=W
  H : PMIOPort  Side=Left
  Q : PMIOPort  Port=2  Side=Left
  W : PMIOPort  Port=3  Side=Right
  T : PMIOPort  Port=4  Side=Right
  connections:
  Qconv12/LConn1 -- Array of Thermal Nodes/LConn12
  Qconv11/LConn1 -- Array of Thermal Nodes/LConn11
  Qconv10/LConn1 -- Array of Thermal Nodes/LConn10
  Qconv9/LConn1 -- Array of Thermal Nodes/LConn9
  Qconv8/LConn1 -- Array of Thermal Nodes/LConn8
  Qconv7/LConn1 -- Array of Thermal Nodes/LConn7
  Qconv6/LConn1 -- Array of Thermal Nodes/LConn6
  Qconv5/LConn1 -- Array of Thermal Nodes/LConn5
  Qconv4/LConn1 -- Array of Thermal Nodes/LConn4
  Qconv3/LConn1 -- Array of Thermal Nodes/LConn3
  Qconv2/LConn1 -- Array of Thermal Nodes/LConn2
  Qconv12/RConn1 -- AirMass/LConn2 -- Qconv11/RConn1 -- Qconv10/RConn1 -- Qconv9/RConn1 -- Qconv8/RConn1 -- Qconv7/RConn1 -- Qconv6/RConn1 -- Qconv5/RConn1 -- Qconv4/RConn1 -- Qconv3/RConn1 -- Qconv2/RConn1 -- Qconv1/RConn1
  Qconv1/LConn1 -- Array of Thermal Nodes/LConn1
  AirMass/RConn1 -- T/RConn1
  Wconv/RConn1 -- W/RConn1
  AirMass/LConn3 -- Wconv/LConn1
  Qfrac/RConn1 -- AirMass/LConn1
  Qfrac/LConn1 -- Q/RConn1
  Array of Thermal Nodes/RConn1 -- H/RConn1

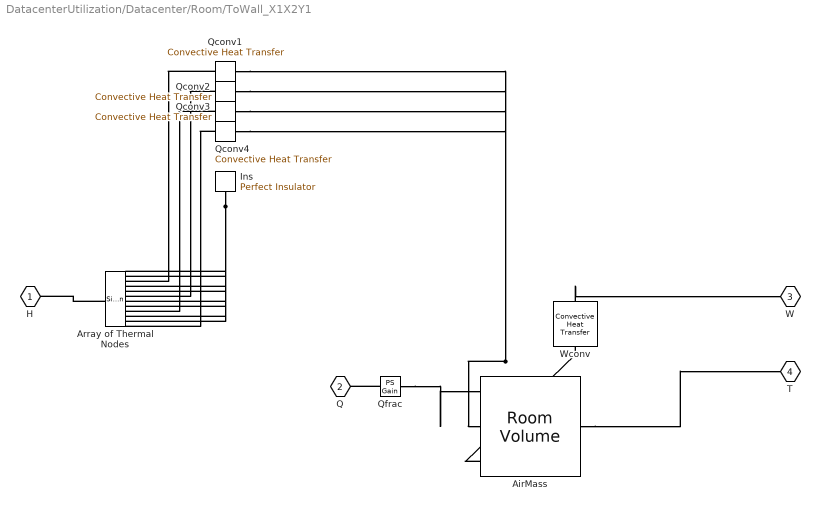
== system DatacenterUtilization/Datacenter/Room/ToWall_X1X2Y1 ==
  AirMass : buildingEnergy_lib/Room Volume  N1=1  N2=1  iniT=300 K  length=12 m  width=0.10667 m  height=8 m
  Array of Thermal Nodes : SimscapeArrayConnection  Domain=foundation.thermal.thermal  ConcatenateDimension=1  NumScalarElements=12
  Ins : fl_lib/Thermal/Thermal Elements/Perfect Insulator  T_specify=off  T_priority=None  T=293.15 K  T_nominal_specify=off  T_nominal_value=1  T_nominal_unit=K
  Qconv{1..4} (4 alike) : fl_lib/Thermal/Thermal Elements/Convective Heat Transfer  thermal_type=foundation.enum.constant_variable.constant  area=12 m^2  heat_tr_coeff=20 W/(K*m^2)  min_heat_tr_coeff=1e-3 W/(K*m^2)  T_specify=off  T_priority=None  T=0 K  T_nominal_specify=off  T_nominal_value=1  T_nominal_unit=K  Q_specify=off  Q_priority=None  Q=0 W  Q_nominal_specify=off  Q_nominal_value=1  Q_nominal_unit=W
  Qfrac : fl_lib/Physical Signals/Functions/PS Gain  gain=0.16667
  Wconv : fl_lib/Thermal/Thermal Elements/Convective Heat Transfer  thermal_type=foundation.enum.constant_variable.constant  area=36 m^2  heat_tr_coeff=20 W/(K*m^2)  min_heat_tr_coeff=1e-3 W/(K*m^2)  T_specify=off  T_priority=None  T=0 K  T_nominal_specify=off  T_nominal_value=1  T_nominal_unit=K  Q_specify=off  Q_priority=None  Q=0 W  Q_nominal_specify=off  Q_nominal_value=1  Q_nominal_unit=W
  H : PMIOPort  Side=Left
  Q : PMIOPort  Port=2  Side=Left
  W : PMIOPort  Port=3  Side=Right
  T : PMIOPort  Port=4  Side=Right
  connections:
  Array of Thermal Nodes/LConn11 -- Array of Thermal Nodes/LConn10 -- Array of Thermal Nodes/LConn8 -- Array of Thermal Nodes/LConn7 -- Array of Thermal Nodes/LConn5 -- Array of Thermal Nodes/LConn4 -- Array of Thermal Nodes/LConn2 -- Ins/LConn1 -- Array of Thermal Nodes/LConn1
  Qconv4/LConn1 -- Array of Thermal Nodes/LConn12
  Qconv3/LConn1 -- Array of Thermal Nodes/LConn9
  Qconv2/LConn1 -- Array of Thermal Nodes/LConn6
  Qconv4/RConn1 -- AirMass/LConn2 -- Qconv3/RConn1 -- Qconv2/RConn1 -- Qconv1/RConn1
  Qconv1/LConn1 -- Array of Thermal Nodes/LConn3
  AirMass/RConn1 -- T/RConn1
  Wconv/RConn1 -- W/RConn1
  AirMass/LConn3 -- Wconv/LConn1
  Qfrac/RConn1 -- AirMass/LConn1
  Qfrac/LConn1 -- Q/RConn1
  Array of Thermal Nodes/RConn1 -- H/RConn1

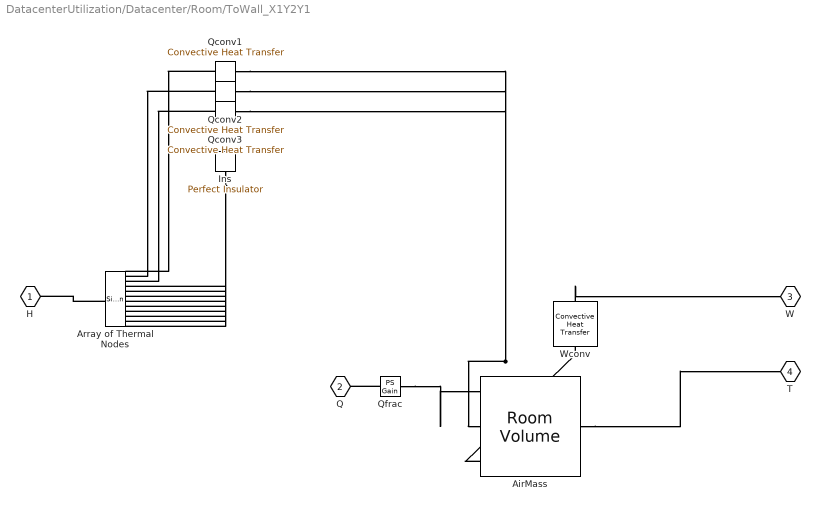
== system DatacenterUtilization/Datacenter/Room/ToWall_X1Y2Y1 ==
  AirMass : buildingEnergy_lib/Room Volume  N1=1  N2=1  iniT=300 K  length=8 m  width=0.10667 m  height=3 m
  Array of Thermal Nodes : SimscapeArrayConnection  Domain=foundation.thermal.thermal  ConcatenateDimension=1  NumScalarElements=12
  Ins : fl_lib/Thermal/Thermal Elements/Perfect Insulator  T_specify=off  T_priority=None  T=293.15 K  T_nominal_specify=off  T_nominal_value=1  T_nominal_unit=K
  Qconv1 : fl_lib/Thermal/Thermal Elements/Convective Heat Transfer  thermal_type=foundation.enum.constant_variable.constant  area=6 m^2  heat_tr_coeff=20 W/(K*m^2)  min_heat_tr_coeff=1e-3 W/(K*m^2)  T_specify=off  T_priority=None  T=0 K  T_nominal_specify=off  T_nominal_value=1  T_nominal_unit=K  Q_specify=off  Q_priority=None  Q=0 W  Q_nominal_specify=off  Q_nominal_value=1  Q_nominal_unit=W
  Qconv2 : fl_lib/Thermal/Thermal Elements/Convective Heat Transfer  thermal_type=foundation.enum.constant_variable.constant  area=6 m^2  heat_tr_coeff=20 W/(K*m^2)  min_heat_tr_coeff=1e-3 W/(K*m^2)  T_specify=off  T_priority=None  T=0 K  T_nominal_specify=off  T_nominal_value=1  T_nominal_unit=K  Q_specify=off  Q_priority=None  Q=0 W  Q_nominal_specify=off  Q_nominal_value=1  Q_nominal_unit=W
  Qconv3 : fl_lib/Thermal/Thermal Elements/Convective Heat Transfer  thermal_type=foundation.enum.constant_variable.constant  area=6 m^2  heat_tr_coeff=20 W/(K*m^2)  min_heat_tr_coeff=1e-3 W/(K*m^2)  T_specify=off  T_priority=None  T=0 K  T_nominal_specify=off  T_nominal_value=1  T_nominal_unit=K  Q_specify=off  Q_priority=None  Q=0 W  Q_nominal_specify=off  Q_nominal_value=1  Q_nominal_unit=W
  Qfrac : fl_lib/Physical Signals/Functions/PS Gain  gain=0.11111
  Wconv : fl_lib/Thermal/Thermal Elements/Convective Heat Transfer  thermal_type=foundation.enum.constant_variable.constant  area=24 m^2  heat_tr_coeff=20 W/(K*m^2)  min_heat_tr_coeff=1e-3 W/(K*m^2)  T_specify=off  T_priority=None  T=0 K  T_nominal_specify=off  T_nominal_value=1  T_nominal_unit=K  Q_specify=off  Q_priority=None  Q=0 W  Q_nominal_specify=off  Q_nominal_value=1  Q_nominal_unit=W
  H : PMIOPort  Side=Left
  Q : PMIOPort  Port=2  Side=Left
  W : PMIOPort  Port=3  Side=Right
  T : PMIOPort  Port=4  Side=Right
  connections:
  Array of Thermal Nodes/LConn12 -- Array of Thermal Nodes/LConn11 -- Array of Thermal Nodes/LConn10 -- Array of Thermal Nodes/LConn9 -- Array of Thermal Nodes/LConn8 -- Array of Thermal Nodes/LConn7 -- Array of Thermal Nodes/LConn6 -- Array of Thermal Nodes/LConn5 -- Ins/LConn1 -- Array of Thermal Nodes/LConn4
  Qconv3/LConn1 -- Array of Thermal Nodes/LConn3
  Qconv2/LConn1 -- Array of Thermal Nodes/LConn2
  Qconv3/RConn1 -- AirMass/LConn2 -- Qconv2/RConn1 -- Qconv1/RConn1
  Qconv1/LConn1 -- Array of Thermal Nodes/LConn1
  AirMass/RConn1 -- T/RConn1
  Wconv/RConn1 -- W/RConn1
  AirMass/LConn3 -- Wconv/LConn1
  Qfrac/RConn1 -- AirMass/LConn1
  Qfrac/LConn1 -- Q/RConn1
  Array of Thermal Nodes/RConn1 -- H/RConn1

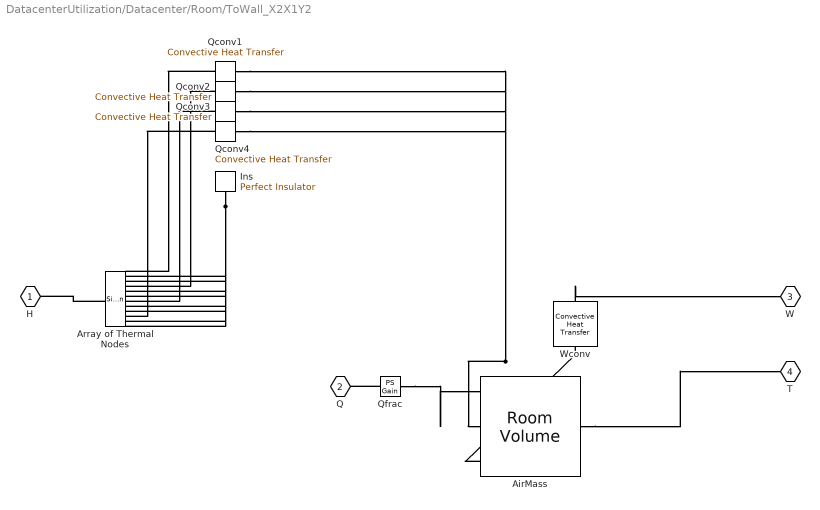
== system DatacenterUtilization/Datacenter/Room/ToWall_X2X1Y2 ==
  AirMass : buildingEnergy_lib/Room Volume  N1=1  N2=1  iniT=300 K  length=12 m  width=0.10667 m  height=3 m
  Array of Thermal Nodes : SimscapeArrayConnection  Domain=foundation.thermal.thermal  ConcatenateDimension=1  NumScalarElements=12
  Ins : fl_lib/Thermal/Thermal Elements/Perfect Insulator  T_specify=off  T_priority=None  T=293.15 K  T_nominal_specify=off  T_nominal_value=1  T_nominal_unit=K
  Qconv{1..4} (4 alike) : fl_lib/Thermal/Thermal Elements/Convective Heat Transfer  thermal_type=foundation.enum.constant_variable.constant  area=12 m^2  heat_tr_coeff=20 W/(K*m^2)  min_heat_tr_coeff=1e-3 W/(K*m^2)  T_specify=off  T_priority=None  T=0 K  T_nominal_specify=off  T_nominal_value=1  T_nominal_unit=K  Q_specify=off  Q_priority=None  Q=0 W  Q_nominal_specify=off  Q_nominal_value=1  Q_nominal_unit=W
  Qfrac : fl_lib/Physical Signals/Functions/PS Gain  gain=0.16667
  Wconv : fl_lib/Thermal/Thermal Elements/Convective Heat Transfer  thermal_type=foundation.enum.constant_variable.constant  area=36 m^2  heat_tr_coeff=20 W/(K*m^2)  min_heat_tr_coeff=1e-3 W/(K*m^2)  T_specify=off  T_priority=None  T=0 K  T_nominal_specify=off  T_nominal_value=1  T_nominal_unit=K  Q_specify=off  Q_priority=None  Q=0 W  Q_nominal_specify=off  Q_nominal_value=1  Q_nominal_unit=W
  H : PMIOPort  Side=Left
  Q : PMIOPort  Port=2  Side=Left
  W : PMIOPort  Port=3  Side=Right
  T : PMIOPort  Port=4  Side=Right
  connections:
  Array of Thermal Nodes/LConn12 -- Array of Thermal Nodes/LConn11 -- Array of Thermal Nodes/LConn9 -- Array of Thermal Nodes/LConn8 -- Array of Thermal Nodes/LConn6 -- Array of Thermal Nodes/LConn5 -- Array of Thermal Nodes/LConn3 -- Ins/LConn1 -- Array of Thermal Nodes/LConn2
  Qconv4/LConn1 -- Array of Thermal Nodes/LConn10
  Qconv3/LConn1 -- Array of Thermal Nodes/LConn7
  Qconv2/LConn1 -- Array of Thermal Nodes/LConn4
  Qconv4/RConn1 -- AirMass/LConn2 -- Qconv3/RConn1 -- Qconv2/RConn1 -- Qconv1/RConn1
  Qconv1/LConn1 -- Array of Thermal Nodes/LConn1
  AirMass/RConn1 -- T/RConn1
  Wconv/RConn1 -- W/RConn1
  AirMass/LConn3 -- Wconv/LConn1
  Qfrac/RConn1 -- AirMass/LConn1
  Qfrac/LConn1 -- Q/RConn1
  Array of Thermal Nodes/RConn1 -- H/RConn1

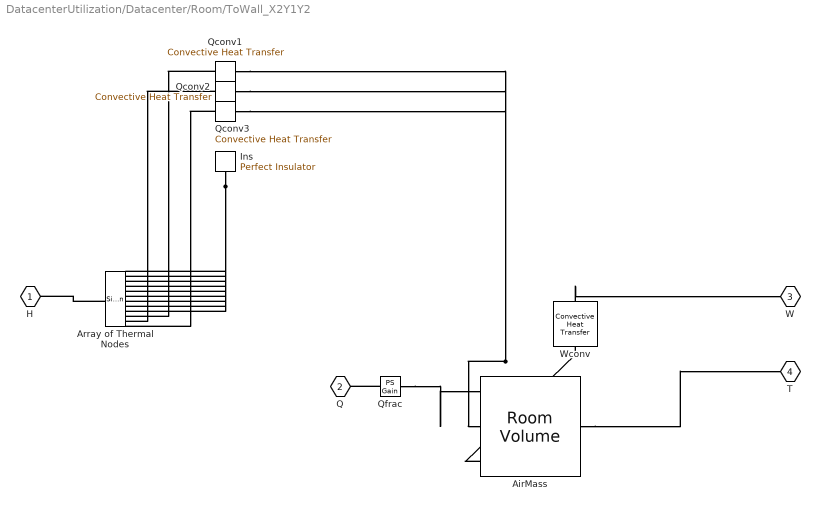
== system DatacenterUtilization/Datacenter/Room/ToWall_X2Y1Y2 ==
  AirMass : buildingEnergy_lib/Room Volume  N1=1  N2=1  iniT=300 K  length=8 m  width=0.10667 m  height=3 m
  Array of Thermal Nodes : SimscapeArrayConnection  Domain=foundation.thermal.thermal  ConcatenateDimension=1  NumScalarElements=12
  Ins : fl_lib/Thermal/Thermal Elements/Perfect Insulator  T_specify=off  T_priority=None  T=293.15 K  T_nominal_specify=off  T_nominal_value=1  T_nominal_unit=K
  Qconv1 : fl_lib/Thermal/Thermal Elements/Convective Heat Transfer  thermal_type=foundation.enum.constant_variable.constant  area=6 m^2  heat_tr_coeff=20 W/(K*m^2)  min_heat_tr_coeff=1e-3 W/(K*m^2)  T_specify=off  T_priority=None  T=0 K  T_nominal_specify=off  T_nominal_value=1  T_nominal_unit=K  Q_specify=off  Q_priority=None  Q=0 W  Q_nominal_specify=off  Q_nominal_value=1  Q_nominal_unit=W
  Qconv2 : fl_lib/Thermal/Thermal Elements/Convective Heat Transfer  thermal_type=foundation.enum.constant_variable.constant  area=6 m^2  heat_tr_coeff=20 W/(K*m^2)  min_heat_tr_coeff=1e-3 W/(K*m^2)  T_specify=off  T_priority=None  T=0 K  T_nominal_specify=off  T_nominal_value=1  T_nominal_unit=K  Q_specify=off  Q_priority=None  Q=0 W  Q_nominal_specify=off  Q_nominal_value=1  Q_nominal_unit=W
  Qconv3 : fl_lib/Thermal/Thermal Elements/Convective Heat Transfer  thermal_type=foundation.enum.constant_variable.constant  area=6 m^2  heat_tr_coeff=20 W/(K*m^2)  min_heat_tr_coeff=1e-3 W/(K*m^2)  T_specify=off  T_priority=None  T=0 K  T_nominal_specify=off  T_nominal_value=1  T_nominal_unit=K  Q_specify=off  Q_priority=None  Q=0 W  Q_nominal_specify=off  Q_nominal_value=1  Q_nominal_unit=W
  Qfrac : fl_lib/Physical Signals/Functions/PS Gain  gain=0.11111
  Wconv : fl_lib/Thermal/Thermal Elements/Convective Heat Transfer  thermal_type=foundation.enum.constant_variable.constant  area=24 m^2  heat_tr_coeff=20 W/(K*m^2)  min_heat_tr_coeff=1e-3 W/(K*m^2)  T_specify=off  T_priority=None  T=0 K  T_nominal_specify=off  T_nominal_value=1  T_nominal_unit=K  Q_specify=off  Q_priority=None  Q=0 W  Q_nominal_specify=off  Q_nominal_value=1  Q_nominal_unit=W
  H : PMIOPort  Side=Left
  Q : PMIOPort  Port=2  Side=Left
  W : PMIOPort  Port=3  Side=Right
  T : PMIOPort  Port=4  Side=Right
  connections:
  Array of Thermal Nodes/LConn9 -- Array of Thermal Nodes/LConn8 -- Array of Thermal Nodes/LConn7 -- Array of Thermal Nodes/LConn6 -- Array of Thermal Nodes/LConn5 -- Array of Thermal Nodes/LConn4 -- Array of Thermal Nodes/LConn3 -- Array of Thermal Nodes/LConn2 -- Ins/LConn1 -- Array of Thermal Nodes/LConn1
  Qconv3/LConn1 -- Array of Thermal Nodes/LConn12
  Qconv2/LConn1 -- Array of Thermal Nodes/LConn11
  Qconv3/RConn1 -- AirMass/LConn2 -- Qconv2/RConn1 -- Qconv1/RConn1
  Qconv1/LConn1 -- Array of Thermal Nodes/LConn10
  AirMass/RConn1 -- T/RConn1
  Wconv/RConn1 -- W/RConn1
  AirMass/LConn3 -- Wconv/LConn1
  Qfrac/RConn1 -- AirMass/LConn1
  Qfrac/LConn1 -- Q/RConn1
  Array of Thermal Nodes/RConn1 -- H/RConn1

== system DatacenterUtilization/Datacenter/Room/Tvec ==
  concat{1..4} (4 alike) : fl_lib/Physical Signals/Functions/PS Concatenate  catColumns=true
  1 : PMIOPort  Side=Left
  2 : PMIOPort  Port=2  Side=Left
  3 : PMIOPort  Port=3  Side=Left
  4 : PMIOPort  Port=4  Side=Left
  5 : PMIOPort  Port=5  Side=Left
  v : PMIOPort  Port=6  Side=Right
  connections:
  concat4/RConn1 -- v/RConn1
  5/RConn1 -- concat4/LConn2
  concat3/RConn1 -- concat4/LConn1
  4/RConn1 -- concat3/LConn2
  concat2/RConn1 -- concat3/LConn1
  3/RConn1 -- concat2/LConn2
  concat1/RConn1 -- concat2/LConn1
  2/RConn1 -- concat1/LConn2
  1/RConn1 -- concat1/LConn1

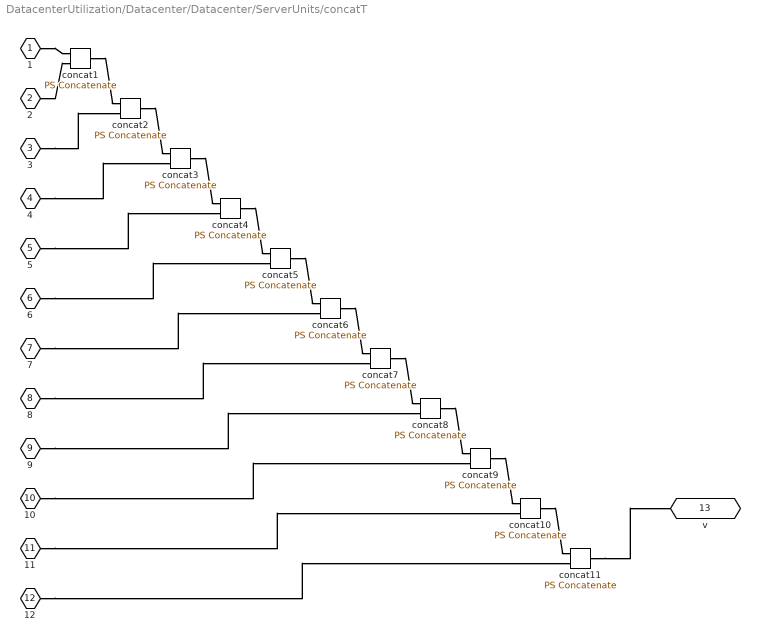
== system DatacenterUtilization/Datacenter/Datacenter/ServerUnits/concatT ==
  concat{1..11} (11 alike) : fl_lib/Physical Signals/Functions/PS Concatenate  catColumns=true
  1 : PMIOPort  Side=Left
  2 : PMIOPort  Port=2  Side=Left
  3 : PMIOPort  Port=3  Side=Left
  4 : PMIOPort  Port=4  Side=Left
  5 : PMIOPort  Port=5  Side=Left
  6 : PMIOPort  Port=6  Side=Left
  7 : PMIOPort  Port=7  Side=Left
  8 : PMIOPort  Port=8  Side=Left
  9 : PMIOPort  Port=9  Side=Left
  10 : PMIOPort  Port=10  Side=Left
  11 : PMIOPort  Port=11  Side=Left
  12 : PMIOPort  Port=12  Side=Left
  v : PMIOPort  Port=13  Side=Right
  connections:
  concat11/RConn1 -- v/RConn1
  12/RConn1 -- concat11/LConn2
  concat10/RConn1 -- concat11/LConn1
  11/RConn1 -- concat10/LConn2
  concat9/RConn1 -- concat10/LConn1
  10/RConn1 -- concat9/LConn2
  concat8/RConn1 -- concat9/LConn1
  9/RConn1 -- concat8/LConn2
  concat7/RConn1 -- concat8/LConn1
  8/RConn1 -- concat7/LConn2
  concat6/RConn1 -- concat7/LConn1
  7/RConn1 -- concat6/LConn2
  concat5/RConn1 -- concat6/LConn1
  6/RConn1 -- concat5/LConn2
  concat4/RConn1 -- concat5/LConn1
  5/RConn1 -- concat4/LConn2
  concat3/RConn1 -- concat4/LConn1
  4/RConn1 -- concat3/LConn2
  concat2/RConn1 -- concat3/LConn1
  3/RConn1 -- concat2/LConn2
  concat1/RConn1 -- concat2/LConn1
  2/RConn1 -- concat1/LConn2
  1/RConn1 -- concat1/LConn1
